simulink model "Escooter"  (R2021b)
settings: Solver=VariableStepAuto  StartTime=0.0  StopTime=10.0  RelTol=1e-3
settings Model: Creator=mariotilocca  LastModifiedBy=mariotilocca

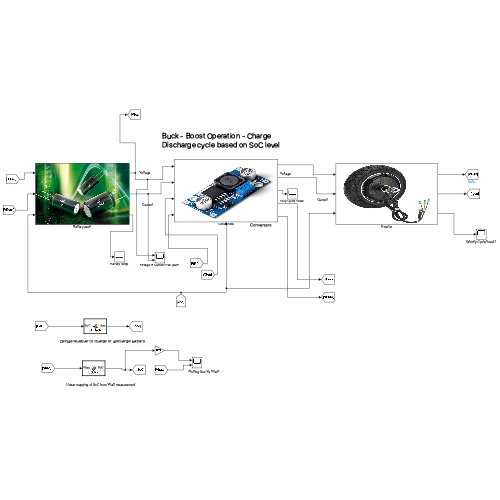
[thumbnail: Simulink's stored preview of the top-level diagram]
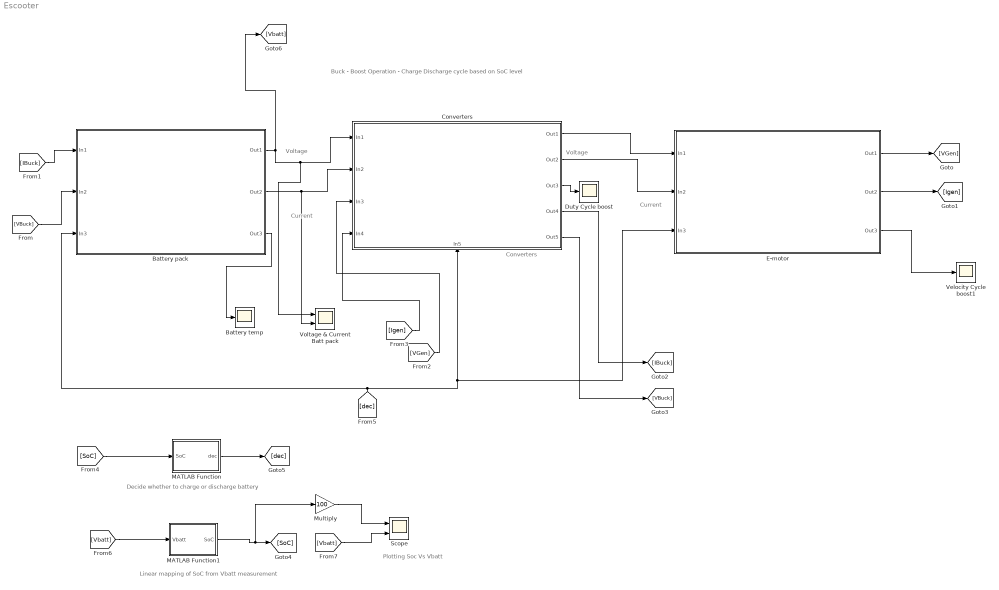
== system Escooter ==
  note: Linear mapping of SoC from Vbatt measurement
  note: Plotting Soc Vs Vbatt
  note: Converters
  note: Decide whether to charge or discharge battery
  note: Buck - Boost Operation - Charge Discharge cycle based on SoC level
  note: Current
  note: Voltage
  note: Current
  note: Voltage
  Battery pack : Subsystem
      mask Display: image('$imagefile'); % Use "Edit Image" on toolstrip to change.
  Battery temp : Scope
  Converters : Subsystem
      settings: PortSchema="{\"entries\":[{\"content\":{\"sides\":[{\"content\":{\"connectorIds\":[\"In1\",\"In2\",\"In3\",\"In4\"]},\"type\":\"ConnectorPlacement.EquallySpacedRectSide\",\"uuid\":\"7e508308-e2f2-4651-b57f-da42e26750df\"},{\"content\":{\"connectorIds\":[\"Out1\",\"Out2\",\"Out3\",\"Out4\",\"Out5\"],\"side\":\"RIGHT\"},\"type\":\"ConnectorPlacement.EquallySpacedRectSide\",\"uuid\":\"a1412a75-01de-4999-bb18-d04890b359be\"},{\"content\":{\"connectorIds\":[],\"side\":\"TOP\"},\"type\":\"ConnectorPlacement.EquallySpacedRectSide\",\"uuid\":\"83fda1a8-b1f7-4fe4-97ce-e68a2dd74e4b\"},{\"content\":{\"connectorIds\":[\"In5\"],\"side\":\"BOTTOM\"},\"type\":\"ConnectorPlacement.EquallySpacedRectSide\",\"uuid\":\"2f960903-1466-4d86-860b-6a835f176349\"}]},\"type\":\"ConnectorPlacement.EquallySpacedConnector\",\"uuid\":\"b0a48f2b-771c-4d63-858c-c6acb924cfbd\"}],\"packageUris\":[\"http://schema.mathworks.com/mf0/Connector/R2020b\"],\"version\":\"1.0\"}"
      mask Display: image('$imagefile'); % Use "Edit Image" on toolstrip to change.
  Duty Cycle boost : Scope
  E-motor : Subsystem
      mask Display: image('$imagefile'); % Use "Edit Image" on toolstrip to change.
  MATLAB Function : MATLAB Function  TreatAsAtomicUnit=on
  MATLAB Function1 : MATLAB Function  TreatAsAtomicUnit=on
  Multiply : Gain  Gain=100
  Scope : Scope  NumInputPorts=2
  Velocity Cycle boost1 : Scope
  "Voltage & Current Batt pack " : Scope  NumInputPorts=2
  wires:
  Converters/1(Out1) -> E-motor/1(In1)
  Converters/2(Out2) -> E-motor/2(In2)
  Battery pack/1(Out1) -> [Vbatt], "Voltage & Current Batt pack "/1, Converters/1(In1)
  Battery pack/2(Out2) -> "Voltage & Current Batt pack "/2, Converters/2(In2)
  Converters/3(Out3) -> Duty Cycle boost/1
  Battery pack/3(Out3) -> Battery temp/1
  E-motor/3(Out3) -> Velocity Cycle boost1/1
  E-motor/1(Out1) -> [VGen]
  [VGen] -> Converters/3(In3)
  E-motor/2(Out2) -> [Igen]
  [Igen] -> Converters/4(In4)
  Converters/4(Out4) -> [IBuck]
  [IBuck] -> Battery pack/1(In1)
  Converters/5(Out5) -> [VBuck]
  [VBuck] -> Battery pack/2(In2)
  [SoC] -> MATLAB Function/1(SoC)
  MATLAB Function/1(dec) -> [dec]
  [dec] -> E-motor/3(In3), Converters/5(In5), Battery pack/3(In3)
  MATLAB Function1/1(SoC) -> Multiply/1, [SoC]
  [Vbatt] -> MATLAB Function1/1(Vbatt)
  [Vbatt] -> Scope/2
  Multiply/1 -> Scope/1

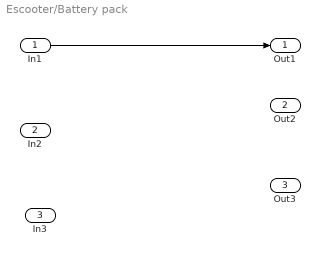
== system Escooter/Battery pack ==
  In1 : Inport
  In2 : Inport  Port=2
  In3 : Inport  Port=3
  Out1 : Outport
  Out2 : Outport  Port=2
  Out3 : Outport  Port=3
  wires:
  In1/1 -> Out1/1

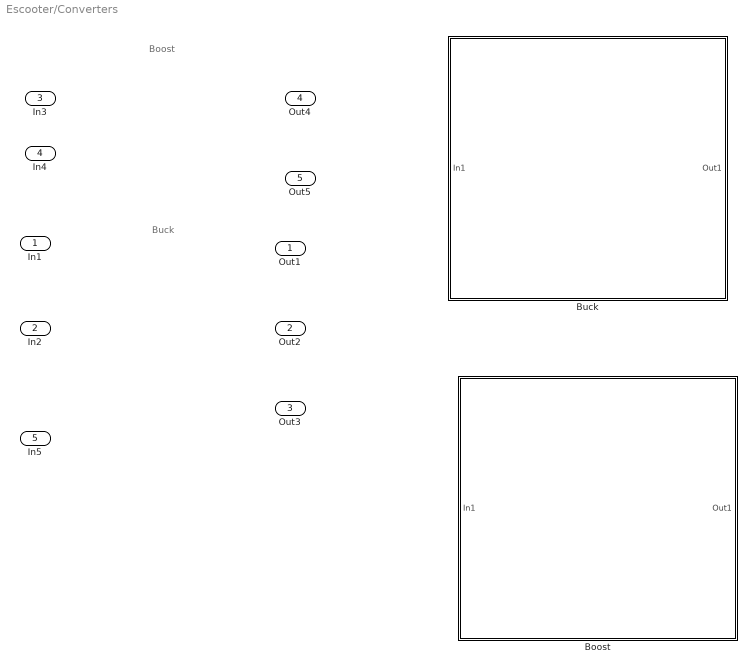
== system Escooter/Converters ==
  note: Buck
  note: Boost
  In1 : Inport
  In2 : Inport  Port=2
  In3 : Inport  Port=3
  In4 : Inport  Port=4
  In5 : Inport  Port=5
  Boost : Subsystem
  Buck : Subsystem
  Out1 : Outport
  Out2 : Outport  Port=2
  Out3 : Outport  Port=3
  Out4 : Outport  Port=4
  Out5 : Outport  Port=5

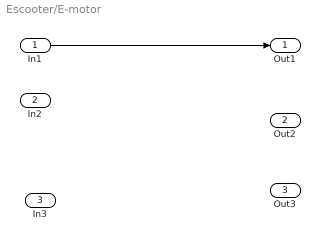
== system Escooter/E-motor ==
  In1 : Inport
  In2 : Inport  Port=2
  In3 : Inport  Port=3
  Out1 : Outport
  Out2 : Outport  Port=2
  Out3 : Outport  Port=3
  wires:
  In1/1 -> Out1/1

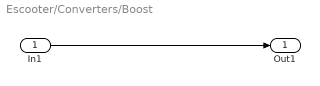
== system Escooter/Converters/Boost ==
  In1 : Inport
  Out1 : Outport
  wires:
  In1/1 -> Out1/1

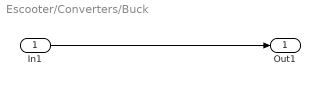
== system Escooter/Converters/Buck ==
  In1 : Inport
  Out1 : Outport
  wires:
  In1/1 -> Out1/1

== matlab function Escooter/MATLAB Function ==
  data: SoC input; dec output
function dec = ChDsch(SoC)


if SoC < 0.05

    dec = 1 ; % discharge 

elseif SoC > 0.05 && SoC == 1
    dec = 2; % charge 

end 


end

== matlab function Escooter/MATLAB Function1 ==
  data: Vbatt input; SoC output
function SoC = SoCalc(Vbatt)

minV = 22;  % TODO -- Load config file for flexible number of  batt cells 
maxV = 38; 

% Linear mapping of SoC 

scaleV = 1/(maxV - minV);
offsetV = -minV * scaleV; 

SoC = Vbatt * scaleV + offsetV ; 

end
